simulink model "BFSKbackup"  (R2018b)
settings: Solver=VariableStepAuto  StartTime=0.0  StopTime=160  RelTol=1e-3
libraries: dsparch4 x6, commsink2 x3, commrandsrc3 x1, commchan3 x1
settings Model: Creator=lance  LastModifiedBy=lance

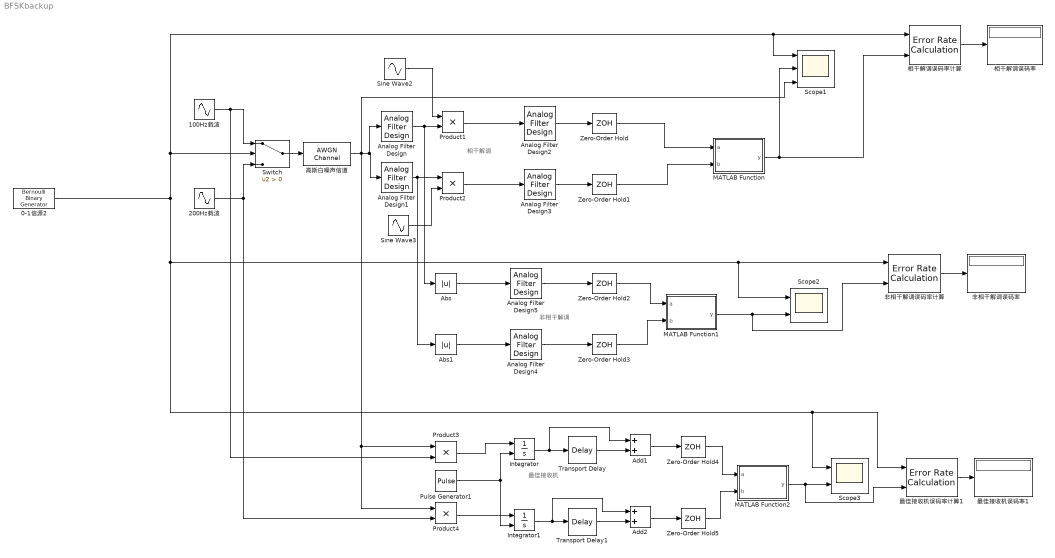
== system BFSKbackup ==
  note: 非相干解调
  note: 相干解调
  note: 最佳接收机
  0-1信源2 : commrandsrc3/Bernoulli Binary Generator  ProbabilityOfZero=0.5  SeedSource=Auto  Seed=61  SampleTime=0.2  SamplesPerFrame=1  OutputDataType=double  SimulateUsing=Interpreted execution
  100Hz载波 : Sin  Frequency=100*2*pi  SampleTime=0.0001
  200Hz载波 : Sin  Frequency=200*2*pi  SampleTime=0.0001
  Abs : Abs
  Abs1 : Abs
  Add1 : Sum
  Add2 : Sum
  Analog Filter Design : dsparch4/Analog Filter Design  method=Butterworth  filttype=Bandpass  N=8  Wlo=90*2*pi  Whi=110*2*pi  Rp=2  Rs=40
  Analog Filter Design1 : dsparch4/Analog Filter Design  method=Butterworth  filttype=Bandpass  N=8  Wlo=190*2*pi  Whi=210*2*pi  Rp=2  Rs=40
  Analog Filter Design{2..5} (4 alike) : dsparch4/Analog Filter Design  method=Butterworth  filttype=Lowpass  N=8  Wlo=10*pi  Whi=103*2*pi  Rp=2  Rs=40
  Integrator : Integrator  ExternalReset=rising
  Integrator1 : Integrator  ExternalReset=rising
  MATLAB Function : MATLAB Function  TreatAsAtomicUnit=on
  MATLAB Function1 : MATLAB Function  TreatAsAtomicUnit=on
  MATLAB Function2 : MATLAB Function  TreatAsAtomicUnit=on
  Product{1..4} (4 alike) : Product
  Pulse Generator1 : DiscretePulseGenerator  PulseType=Time based  Period=0.2
  Scope1 : Scope  NumInputPorts=3
  Scope2 : Scope  NumInputPorts=2
  Scope3 : Scope  NumInputPorts=2
  Sine Wave2 : Sin  Frequency=100*2*pi  SampleTime=0.0001
  Sine Wave3 : Sin  Frequency=200*2*pi  SampleTime=0.0001
  Switch : Switch  Criteria=u2 > Threshold
  Transport Delay : TransportDelay  DelayTime=0.02
  Transport Delay1 : TransportDelay  DelayTime=0.02
  Zero-Order Hold{,1..5} (6 alike) : ZeroOrderHold  SampleTime=0.2
  最佳接收机误码率1 : Display
  最佳接收机误码率计算1 : commsink2/Error Rate Calculation  N=1  st_delay=0  cp_mode=Entire frame  subframe=[]  PMode=Port  WsName=ErrorVec  RsMode2=off  stop=off  numErr=100  maxBits=1e6
  相干解调误码率 : Display
  "相干解调误码率计算 " : commsink2/Error Rate Calculation  N=2  st_delay=0  cp_mode=Entire frame  subframe=[]  PMode=Port  WsName=ErrorVec  RsMode2=off  stop=off  numErr=100  maxBits=1e6
  非相干解调误码率 : Display
  非相干解调误码率计算 : commsink2/Error Rate Calculation  N=2  st_delay=0  cp_mode=Entire frame  subframe=[]  PMode=Port  WsName=ErrorVec  RsMode2=off  stop=off  numErr=100  maxBits=1e6
  "高斯白噪声信道 " : commchan3/AWGN Channel  InputProcessing=Columns as channels (frame based)  seed=67  noiseMode="Signal to noise ratio  (SNR)"  EbNodB=1  EsNodB=10  SNRdB=-18  bitsPerSym=1  Ps=1  Tsym=1  variance=1
  wires:
  100Hz载波/1 -> Product3/2, Switch/1
  200Hz载波/1 -> Switch/3, Product4/2
  Sine Wave2/1 -> Product1/1
  Analog Filter Design/1 -> Abs/1, Product1/2
  Sine Wave3/1 -> Product2/2
  Analog Filter Design1/1 -> Abs1/1, Product2/1
  Product1/1 -> Analog Filter Design2/1
  Product2/1 -> Analog Filter Design3/1
  Analog Filter Design3/1 -> Zero-Order Hold1/1
  Analog Filter Design2/1 -> Zero-Order Hold/1
  "相干解调误码率计算 "/1 -> 相干解调误码率/1
  Zero-Order Hold/1 -> MATLAB Function/1(a)
  Zero-Order Hold1/1 -> MATLAB Function/2(b)
  MATLAB Function/1(y) -> Scope1/2, "相干解调误码率计算 "/2
  Switch/1 -> "高斯白噪声信道 "/1
  "高斯白噪声信道 "/1 -> Product4/1, Product3/1, Analog Filter Design1/1, Analog Filter Design/1, Scope1/3
  Abs/1 -> Analog Filter Design5/1
  Abs1/1 -> Analog Filter Design4/1
  Analog Filter Design5/1 -> Zero-Order Hold2/1
  Analog Filter Design4/1 -> Zero-Order Hold3/1
  Zero-Order Hold2/1 -> MATLAB Function1/1(a)
  Zero-Order Hold3/1 -> MATLAB Function1/2(b)
  MATLAB Function1/1(y) -> Scope2/2, 非相干解调误码率计算/2
  非相干解调误码率计算/1 -> 非相干解调误码率/1
  Product3/1 -> Integrator/1
  Pulse Generator1/1 -> Integrator1/2, Integrator/2
  Product4/1 -> Integrator1/1
  Integrator1/1 -> Add2/1, Transport Delay1/1
  Integrator/1 -> Add1/1, Transport Delay/1
  Transport Delay/1 -> Add1/2
  Transport Delay1/1 -> Add2/2
  Zero-Order Hold4/1 -> MATLAB Function2/1(a)
  Zero-Order Hold5/1 -> MATLAB Function2/2(b)
  Add1/1 -> Zero-Order Hold4/1
  Add2/1 -> Zero-Order Hold5/1
  最佳接收机误码率计算1/1 -> 最佳接收机误码率1/1
  MATLAB Function2/1(y) -> 最佳接收机误码率计算1/2, Scope3/2
  0-1信源2/1 -> 非相干解调误码率计算/1, Scope2/1, Scope3/1, 最佳接收机误码率计算1/1, Switch/2, "相干解调误码率计算 "/1, Scope1/1

== matlab function BFSKbackup/MATLAB Function1 ==
  data: a input; y output; b input
function y = fcn(a, b)
if(a>b)
    y=1;
else
    y=0;
end

== matlab function BFSKbackup/MATLAB Function ==
  data: a input; y output; b input
function y = fcn(a, b)
if(a>b)
    y=1;
else
    y=0;
end

== matlab function BFSKbackup/MATLAB Function2 ==
  data: a input; y output; b input
function y = fcn(a, b)
if(a>b)
    y=1;
else
    y=0;
end
